simulink model "week1_problem8"  (R2020b)
settings: Solver=VariableStepAuto  StartTime=0.0  StopTime=10.0  RelTol=1e-3
settings Model: Creator=omkar  LastModifiedBy=omkar

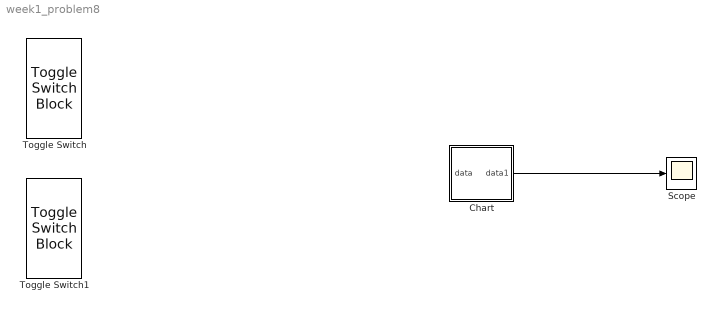
== system week1_problem8 ==
  Chart : Stateflow chart  TreatAsAtomicUnit=on
  Scope : Scope
  Toggle Switch : ToggleSwitchBlock
      settings: Values={{'Off', 'On'}, [0 1]}
  Toggle Switch1 : ToggleSwitchBlock
      settings: Values={{'Off', 'On'}, [0 2]}
  wires:
  Chart/1(data1) -> Scope/1

== stateflow chart week1_problem8/Chart ==
  state GroundFloor
  state FirstFloor
  (default) -> GroundFloor
  GroundFloor -> FirstFloor : [Toggle_Switch==1]
  FirstFloor -> GroundFloor : [Toggle_Switch1==2]
  data: data input; data1 output
